simulink model "template_KR3_PreRTHS"  (Simulink 8.2)
settings: Solver=FixedStepDiscrete  StartTime=0.0  StopTime=RunningTime  FixedStep=sample  RelTol=1e-3
undefined symbols (not defined in the file): ElementsStruct, Integrator, NumFreeDOF, RigidLinkMasterMatrix, RigidLinkNo, RigidLinkNodeID, RigidLinkSlaveMatrix, sample, SampleRate, Structure
libraries: HybridFEMLibrary x1
(part 1 of 2)
CloseFcn:
  | rtwprivate ssgencode ModelCloseRequest hybriddaq1dof
settings Model: MinMaxOverflowLogging=ForceOff  Creator=RTMD  LastModifiedBy=Thomas Marullo  BufferReuse=off
settings DataIOCC: LimitDataPoints=off
settings OptimizationCC: BlockReduction=off  OptimizeBlockIOStorage=off  BufferReuse=off  ExpressionFolding=off  LocalBlockOutputs=off  InitFltsAndDblsToZero=on
settings DebuggingCC: SignalResolutionControl=TryResolveAllWithWarning  MultiTaskDSMMsg=warning  FcnCallInpInsideContextMsg=EnableAllAsWarning
settings HardwareCC: ProdIntDivRoundTo=Zero  ProdEndianess=LittleEndian  ProdHWDeviceType=Generic->32-bit x86 compatible
settings SFSimCC: SimParseCustomCode=off
settings RTWCC: SystemTargetFile=xpctarget.tlc  TemplateMakefile=xpc_default_tmf  Description=xPC Target  ProcessScript=xpctarget_make_rtw_hook
settings TargetCC: CodeReplacementLibrary=XPC_BLAS  IsPILTarget=off  ParMdlRefBuildCompliant=on  ConcurrentExecutionCompliant=on  MatFileLogging=on  EnableShiftOperators=on
settings CustomProperty: DataType=string  Value=Real-Time

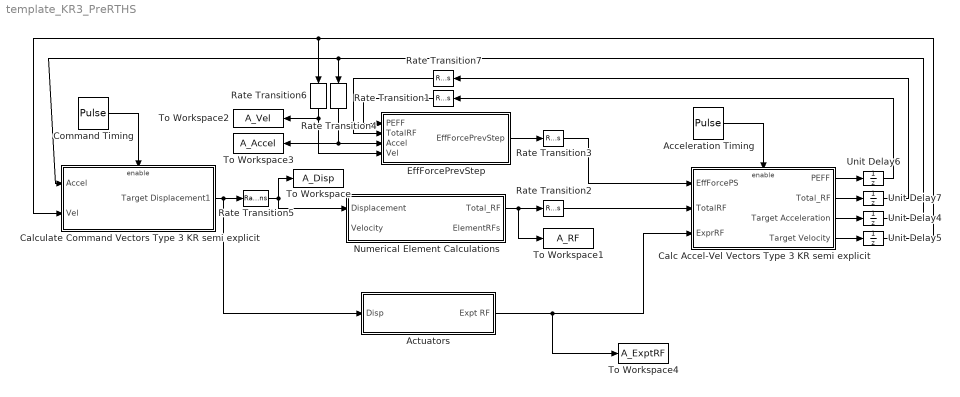
== system template_KR3_PreRTHS ==
  Acceleration Timing : DiscretePulseGenerator  Period=Integrator.Interpolations  PhaseDelay=Integrator.Interpolations-1  SampleTime=sample
  Actuators : Subsystem
  Calc Accel-Vel Vectors Type 3 KR semi explicit : Subsystem
  Calculate Command Vectors Type 3 KR semi explicit : Subsystem  TreatAsAtomicUnit=on  SystemSampleTime=SampleRate
  Command Timing : DiscretePulseGenerator  Period=Integrator.Interpolations  SampleTime=sample
  EffForcePrevStep : Subsystem  TreatAsAtomicUnit=on
  Numerical Element Calculations : MATLAB Function  TreatAsAtomicUnit=on
  Rate Transition{1,4,6..7} (4 alike) : RateTransition  Deterministic=off  X0=-1  OutPortSampleTime=SampleRate
  Rate Transition2 : RateTransition  Deterministic=off  OutPortSampleTime=sample
  Rate Transition3 : RateTransition  Deterministic=off  OutPortSampleTime=sample
  Rate Transition5 : RateTransition  Deterministic=off  OutPortSampleTime=SampleRate
  To Workspace : ToWorkspace  VariableName=A_Disp  SampleTime=-1
  To Workspace1 : ToWorkspace  VariableName=A_RF  SampleTime=-1
  To Workspace2 : ToWorkspace  VariableName=A_Vel  SampleTime=-1
  To Workspace3 : ToWorkspace  VariableName=A_Accel  SampleTime=-1
  To Workspace4 : ToWorkspace  VariableName=A_ExptRF  SampleTime=-1
  Unit Delay{4..7} (4 alike) : UnitDelay  SampleTime=-1
  wires:
  Calc Accel-Vel Vectors Type 3 KR semi explicit/3(Target Acceleration) -> Unit Delay4/1
  Calculate Command Vectors Type 3 KR semi explicit/1(Target Displacement1) -> Actuators/1(Disp), Rate Transition5/1
  Calc Accel-Vel Vectors Type 3 KR semi explicit/4(Target Velocity) -> Unit Delay5/1
  Command Timing/1 -> Calculate Command Vectors Type 3 KR semi explicit/Enable
  Rate Transition2/1 -> Calc Accel-Vel Vectors Type 3 KR semi explicit/2(TotalRF)
  Calc Accel-Vel Vectors Type 3 KR semi explicit/1(PEFF) -> Unit Delay6/1
  EffForcePrevStep/1(EffForcePrevStep) -> Rate Transition3/1
  Rate Transition3/1 -> Calc Accel-Vel Vectors Type 3 KR semi explicit/1(EffForcePS)
  Rate Transition5/1 -> Numerical Element Calculations/1(Displacement), To Workspace/1
  Unit Delay5/1 -> Rate Transition6/1, Calculate Command Vectors Type 3 KR semi explicit/2(Vel)
  Rate Transition1/1 -> EffForcePrevStep/1(PEFF)
  Acceleration Timing/1 -> Calc Accel-Vel Vectors Type 3 KR semi explicit/Enable
  Rate Transition4/1 -> EffForcePrevStep/3(Accel), To Workspace3/1
  Rate Transition6/1 -> EffForcePrevStep/4(Vel), To Workspace2/1
  Calc Accel-Vel Vectors Type 3 KR semi explicit/2(Total_RF) -> Unit Delay7/1
  Rate Transition7/1 -> EffForcePrevStep/2(TotalRF)
  Unit Delay7/1 -> Rate Transition7/1
  Unit Delay6/1 -> Rate Transition1/1
  Unit Delay4/1 -> Rate Transition4/1, Calculate Command Vectors Type 3 KR semi explicit/1(Accel)
  Actuators/1(Expt RF) -> To Workspace4/1, Calc Accel-Vel Vectors Type 3 KR semi explicit/3(ExprRF)
  Numerical Element Calculations/1(Total_RF) -> Rate Transition2/1, To Workspace1/1

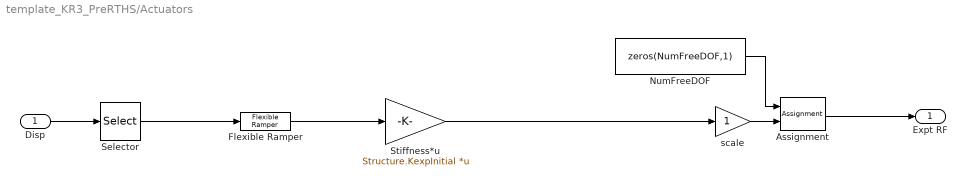
== system template_KR3_PreRTHS/Actuators ==
  Disp : Inport
  Assignment : Assignment  IndexOptions=Index vector (dialog)  Indices=Structure.InterfaceDOF  OutputSizes=1
  Flexible Ramper : HybridFEMLibrary/Flexible Ramper  ramps=Integrator.Interpolations  samplerate=sample  initVal=zeros(size(Structure.InterfaceDOF),1)
  NumFreeDOF : Constant  Value=zeros(NumFreeDOF,1)
  Selector : Selector  InputPortWidth=NumFreeDOF  IndexOptions=Index vector (dialog)  Indices=Structure.InterfaceDOF  OutputSizes=1
  Stiffness*u : Gain  Gain=Structure.KexpInitial  Multiplication=Matrix(K*u) (u vector)
  scale : Gain
  Expt RF : Outport
  wires:
  Disp/1 -> Selector/1
  Selector/1 -> Flexible Ramper/1
  Assignment/1 -> Expt RF/1
  Stiffness*u/1 -> scale/1
  NumFreeDOF/1 -> Assignment/1
  scale/1 -> Assignment/2
  Flexible Ramper/1 -> Stiffness*u/1

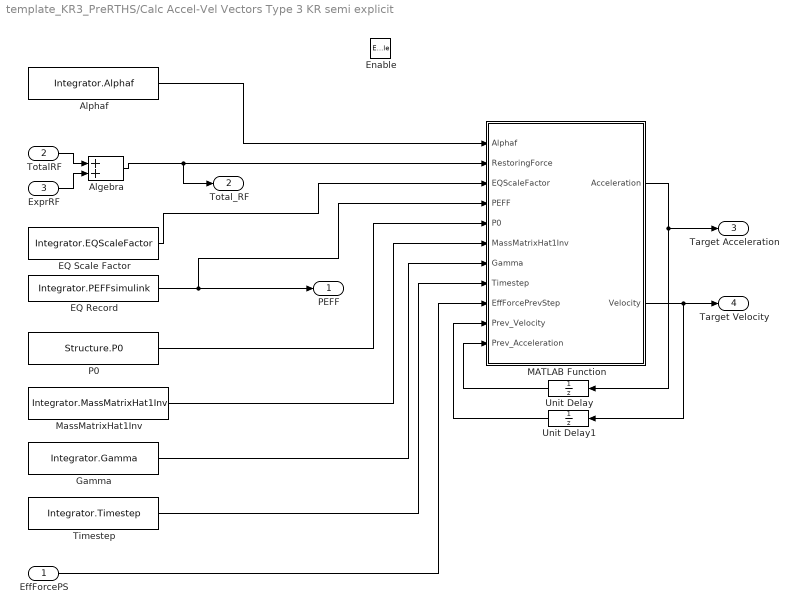
== system template_KR3_PreRTHS/Calc Accel-Vel Vectors Type 3 KR semi explicit ==
  EffForcePS : Inport
  TotalRF : Inport  Port=2
  ExprRF : Inport  Port=3
  Enable : EnablePort
  Algebra : Sum
  Alphaf : Constant  Value=Integrator.Alphaf
  EQ Record : FromWorkspace  VariableName=Integrator.PEFFsimulink  Interpolate=off  OutputAfterFinalValue=Holding final value
  EQ Scale Factor : Constant  Value=Integrator.EQScaleFactor
  Gamma : Constant  Value=Integrator.Gamma
  MATLAB Function : MATLAB Function  TreatAsAtomicUnit=on
  MassMatrixHat1Inv : Constant  Value=Integrator.MassMatrixHat1Inv
  P0 : Constant  Value=Structure.P0
  Timestep : Constant  Value=Integrator.Timestep
  Unit Delay : UnitDelay  SampleTime=-1
  Unit Delay1 : UnitDelay  SampleTime=-1
  PEFF : Outport
  Total_RF : Outport  Port=2
  Target Acceleration : Outport  Port=3
  Target Velocity : Outport  Port=4
  wires:
  EffForcePS/1 -> MATLAB Function/9(EffForcePrevStep)
  Unit Delay1/1 -> MATLAB Function/10(Prev_Velocity)
  Unit Delay/1 -> MATLAB Function/11(Prev_Acceleration)
  Timestep/1 -> MATLAB Function/8(Timestep)
  Gamma/1 -> MATLAB Function/7(Gamma)
  MassMatrixHat1Inv/1 -> MATLAB Function/6(MassMatrixHat1Inv)
  P0/1 -> MATLAB Function/5(P0)
  EQ Scale Factor/1 -> MATLAB Function/3(EQScaleFactor)
  EQ Record/1 -> PEFF/1, MATLAB Function/4(PEFF)
  MATLAB Function/2(Velocity) -> Unit Delay1/1, Target Velocity/1
  Alphaf/1 -> MATLAB Function/1(Alphaf)
  Algebra/1 -> MATLAB Function/2(RestoringForce), Total_RF/1
  ExprRF/1 -> Algebra/2
  TotalRF/1 -> Algebra/1
  MATLAB Function/1(Acceleration) -> Unit Delay/1, Target Acceleration/1

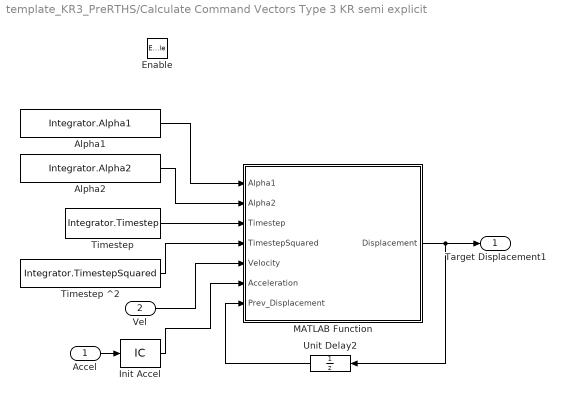
== system template_KR3_PreRTHS/Calculate Command Vectors Type 3 KR semi explicit ==
  Accel : Inport
  Vel : Inport  Port=2
  Enable : EnablePort
  Alpha1 : Constant  Value=Integrator.Alpha1
  Alpha2 : Constant  Value=Integrator.Alpha2
  Init Accel : InitialCondition  Value=Integrator.Acceleration
  MATLAB Function : MATLAB Function  TreatAsAtomicUnit=on
  Timestep : Constant  Value=Integrator.Timestep
  Timestep ^2 : Constant  Value=Integrator.TimestepSquared
  Unit Delay2 : UnitDelay  SampleTime=-1
  Target Displacement1 : Outport
  wires:
  Accel/1 -> Init Accel/1
  MATLAB Function/1(Displacement) -> Target Displacement1/1, Unit Delay2/1
  Unit Delay2/1 -> MATLAB Function/7(Prev_Displacement)
  Alpha1/1 -> MATLAB Function/1(Alpha1)
  Alpha2/1 -> MATLAB Function/2(Alpha2)
  Timestep/1 -> MATLAB Function/3(Timestep)
  Timestep ^2/1 -> MATLAB Function/4(TimestepSquared)
  Vel/1 -> MATLAB Function/5(Velocity)
  Init Accel/1 -> MATLAB Function/6(Acceleration)

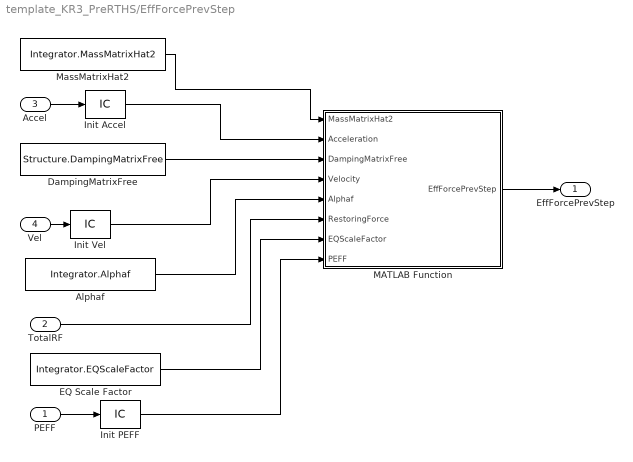
== system template_KR3_PreRTHS/EffForcePrevStep ==
  PEFF : Inport
  TotalRF : Inport  Port=2
  Accel : Inport  Port=3
  Vel : Inport  Port=4
  Alphaf : Constant  Value=Integrator.Alphaf
  DampingMatrixFree : Constant  Value=Structure.DampingMatrixFree
  EQ Scale Factor : Constant  Value=Integrator.EQScaleFactor
  Init Accel : InitialCondition  Value=Integrator.Acceleration
  Init PEFF : InitialCondition  Value=Integrator.PEFF(1,:)
  Init Vel : InitialCondition  Value=Integrator.Velocity
  MATLAB Function : MATLAB Function  TreatAsAtomicUnit=on
  MassMatrixHat2 : Constant  Value=Integrator.MassMatrixHat2
  EffForcePrevStep : Outport
  wires:
  PEFF/1 -> Init PEFF/1
  Vel/1 -> Init Vel/1
  MassMatrixHat2/1 -> MATLAB Function/1(MassMatrixHat2)
  Accel/1 -> Init Accel/1
  Init Accel/1 -> MATLAB Function/2(Acceleration)
  DampingMatrixFree/1 -> MATLAB Function/3(DampingMatrixFree)
  Init Vel/1 -> MATLAB Function/4(Velocity)
  Alphaf/1 -> MATLAB Function/5(Alphaf)
  TotalRF/1 -> MATLAB Function/6(RestoringForce)
  EQ Scale Factor/1 -> MATLAB Function/7(EQScaleFactor)
  Init PEFF/1 -> MATLAB Function/8(PEFF)
  MATLAB Function/1(EffForcePrevStep) -> EffForcePrevStep/1

== matlab function Calculate Command Vectors Type 3 KR semi explicit/MATLAB Function ==
  data: Alpha1 input double; Alpha2 input double; Timestep input double; TimestepSquared input double; Velocity input double; Acceleration input double; Displacement output double; Prev_Displacement input double
function Displacement   = fcn(Alpha1,...
                                Alpha2,...
                                Timestep,...
                                TimestepSquared,...
                                Velocity,...
                                Acceleration,...
                                Prev_Displacement)

Displacement = Prev_Displacement + ...
                    Alpha1 * Timestep * Velocity + ...
                    Alpha2 * TimestepSquared * Acceleration;

== matlab function Calc Accel-Vel Vectors Type 3 KR semi explicit/MATLAB Function ==
  data: Alphaf input double; RestoringForce input double; Acceleration output double; Velocity output double; EQScaleFactor input double; PEFF input double; P0 input double; MassMatrixHat1Inv input double; Gamma input double; Timestep input double; EffForcePrevStep input double; Prev_Velocity input double; Prev_Acceleration input double
function [Acceleration,Velocity] = fcn(Alphaf,...                                                        
                            RestoringForce,...                              
                            EQScaleFactor,...
                            PEFF,...      
                            P0,... 
                            MassMatrixHat1Inv,...
                            Gamma,...
                            Timestep,...
                            EffForcePrevStep,...
                            Prev_Velocity,...
                            Prev_Acceleration)
                                                

Acceleration = MassMatrixHat1Inv * ...
                          ((1 - Alphaf) * (EQScaleFactor * PEFF - ...
                          RestoringForce) - EffForcePrevStep + P0);
                      
Velocity = Prev_Velocity + Timestep * ((1 - Gamma) * Prev_Acceleration + ...
                      Gamma * Acceleration);
